simulink model "Resp18e_updatedPulse"  (Simulink 7.3)
settings: Solver=ode23  StartTime=0.0  StopTime=20  FixedStep=0.01  MaxStep=0.05  RelTol=1e-6
values from neighbouring files (symbols this model uses):
  alpha_CO2_brain = 2.9/1e3*760/P_stp/K_stp    (= 0.00097047576489)    [initialize_parameters.m]
  alpha_CO2_fat = 0.9/K_stp/P_stp    (= 0.000396292281489)    [initialize_parameters.m]
  alpha_CO2_heart = 2.4/1e3*760/P_stp/K_stp    (= 0.00080315235715)    [initialize_parameters.m]
  alpha_CO2_lean = 4.2/1e3*760/P_stp/K_stp    (= 0.00140551662501)    [initialize_parameters.m]
  alpha_CO2_lungtiss_fast = alpha_CO2_lungtiss_fast./0.1333    [initialize_parameters.m]
  alpha_CO2_muscle = 4.2/1e3*760/P_stp/K_stp    (= 0.00140551662501)    [initialize_parameters.m]
  alpha_CO2_other = 3.0/1e3*760/P_stp/K_stp    (= 0.00100394044644)    [initialize_parameters.m]
  alpha_O2_fat = 5*0.024/K_stp/P_stp    (= 5.28389708651e-05)    [initialize_parameters.m]
  alpha_O2_tissue = 0.024/K_stp/P_stp    (= 1.0567794173e-05)    [initialize_parameters.m]
  BOHRF0 = O2_SHIFT - T_BLOOD_M_37 * (0.024 + BOHRF * 0.0147) - BOHRF1 * 7.4    (= -3.552)    [initialize_parameters.m]
  BOHRF1 = BOHRF * (1 - T_BLOOD_M_37 * 0.0065)    (= 0.48)    [initialize_parameters.m]
  C_a_CO2_i = 20.8e-3    (= 0.0208)    [initialize_parameters.m]    (also in resp18e_ic_norm.mat = 0.0202734801806)
  C_a_O2_i = 8.95e-3    (= 0.00895)    [initialize_parameters.m]    (also in resp18e_ic_norm.mat = 0.00918087581167)
  CAP_O2 = 0.01 * CAP_O2    (= 0.201)    [initialize_parameters.m]
  Cardiac_duty_cycle = 40    [initialize_parameters.m]
  Co_CO2_brain = 401*K_Co_CO2/1e3/K_stp    (= 0.0107345869894)    [initialize_parameters.m]
  Co_CO2_heart = 487*K_Co_CO2/1e3/K_stp    (= 0.0130367677403)    [initialize_parameters.m]
  Co_CO2_lean = 342*K_Co_CO2/1e3/K_stp    (= 0.00915518391618)    [initialize_parameters.m]
  Co_CO2_muscle = 342*K_Co_CO2/1e3/K_stp    (= 0.00915518391618)    [initialize_parameters.m]
  Co_CO2_other = 355*K_Co_CO2/1e3/K_stp    (= 0.00950318798317)    [initialize_parameters.m]
  DH2ODS = DH2ODS + 0.007 * HB_MEQ * (HB_MEQ - 9) / (13.5 * (13.5 - 9))    (= 0.00498709726946)    [initialize_parameters.m]
  F_insp_alv_alvds = F_v_alv_deadspace / F_insp_hivq    (= 0.00299401197605)    [initialize_parameters.m]
  F_insp_alv_hivq = F_v_alv_hivq      / F_insp_hivq    (= 0.997005988024)    [initialize_parameters.m]
  F_insp_alv_lovq = F_v_alv_lovq      / F_insp_lovq    (= 0.5)    [initialize_parameters.m]
  F_insp_alv_midvq = F_v_alv_midvq     / F_insp_lovq    (= 0.5)    [initialize_parameters.m]
  F_insp_hivq = F_v_alv_deadspace + F_v_alv_hivq    (= 0.334)    [initialize_parameters.m]
  F_insp_lovq = F_v_alv_midvq     + F_v_alv_lovq    (= 0.666)    [initialize_parameters.m]
  Fi_CO2_param_est = 0.01    [initialize_parameters.m]
  Fi_error = 1e-6    (= 1e-06)    [initialize_parameters.m]
  Fi_N2_mean = 1-(Fi_O2_mean + Fi_N2O_mean)    (= 0.65)    [initialize_parameters.m]
  Fi_O2_mean = 0.35    [initialize_parameters.m]
  Fi_O2_param_est = 0.01    [initialize_parameters.m]
  Fq_brain = 0.114    [initialize_parameters.m]
  Fq_error = 1e-8    (= 1e-08)    [initialize_parameters.m]
  Fq_fat = 0.103    [initialize_parameters.m]
  Fq_heart = 0.041    [initialize_parameters.m]
  Fq_hepatic = 0.069    [initialize_parameters.m]
  Fq_kidneys = 0.215    [initialize_parameters.m]
  Fq_lean = 0.090    (= 0.09)    [initialize_parameters.m]
  Fq_lungs_anatomicalshunt = 0.01    [initialize_parameters.m]
  Fq_lungs_hivq = (1-Fq_lungs_pulmshunt-Fq_lungs_anatomicalshunt)    *F_v_alv_hivq/(F_v_alv_hivq+F_v_alv_midvq+F_v_alv_lovq)    (= 0.3)    [initialize_parameters.m]
  Fq_lungs_lovq = (1-Fq_lungs_pulmshunt-Fq_lungs_anatomicalshunt)    *F_v_alv_lovq/(F_v_alv_hivq+F_v_alv_midvq+F_v_alv_lovq)    (= 0.3)    [initialize_parameters.m]
  Fq_lungs_midvq = (1-Fq_lungs_pulmshunt-Fq_lungs_anatomicalshunt)    *F_v_alv_midvq/(F_v_alv_hivq+F_v_alv_midvq+F_v_alv_lovq)    (= 0.3)    [initialize_parameters.m]
  Fq_lungs_pulmshunt = 0.09    [initialize_parameters.m]
  Fq_muscle = 0.096    [initialize_parameters.m]
  Fq_pershunt = 0.101    [initialize_parameters.m]
  Fq_portal = 0.171    [initialize_parameters.m]
  FRC = 2.2    [initialize_parameters.m]
  H2OB = H2OVC + 0.938 * (1 - VC_74)    (= 0.840191964286)    [initialize_parameters.m]
  k_CO2_lungtiss_fast_alvds = k_CO2_lungtiss_fast*F_v_alv_deadspace    (= 3.63090772693e-07)    [initialize_parameters.m]
  k_CO2_lungtiss_fast_hivq = k_CO2_lungtiss_fast*F_v_alv_hivq    (= 0.000120909227307)    [initialize_parameters.m]
  k_CO2_lungtiss_fast_lovq = k_CO2_lungtiss_fast*F_v_alv_lovq    (= 0.000120909227307)    [initialize_parameters.m]
  k_CO2_lungtiss_fast_midvq = k_CO2_lungtiss_fast*F_v_alv_midvq    (= 0.000120909227307)    [initialize_parameters.m]
  k_CO2_lungtiss_slow_alvds = k_CO2_lungtiss_slow*F_v_alv_deadspace    (= 4.95123780945e-09)    [initialize_parameters.m]
  k_CO2_lungtiss_slow_hivq = k_CO2_lungtiss_slow*F_v_alv_hivq    (= 1.64876219055e-06)    [initialize_parameters.m]
  k_CO2_lungtiss_slow_lovq = k_CO2_lungtiss_slow*F_v_alv_lovq    (= 1.64876219055e-06)    [initialize_parameters.m]
  k_CO2_lungtiss_slow_midvq = k_CO2_lungtiss_slow*F_v_alv_midvq    (= 1.64876219055e-06)    [initialize_parameters.m]
  K_diff_CO2_hivq = K_diff_CO2*F_v_alv_hivq    (= 0.0014985)    [initialize_parameters.m]
  K_diff_CO2_lovq = K_diff_CO2*F_v_alv_lovq    (= 0.0014985)    [initialize_parameters.m]
  K_diff_CO2_midvq = K_diff_CO2*F_v_alv_midvq    (= 0.0014985)    [initialize_parameters.m]
  K_diff_O2_hivq = K_diff_O2*F_v_alv_hivq    (= 7.326e-05)    [initialize_parameters.m]
  K_diff_O2_lovq = K_diff_O2*F_v_alv_lovq    (= 7.326e-05)    [initialize_parameters.m]
  K_diff_O2_midvq = K_diff_O2*F_v_alv_midvq    (= 7.326e-05)    [initialize_parameters.m]
  K_exp_alv_alvds = 1/1    (= 1)    [initialize_parameters.m]
  K_exp_alv_hivq = 1/1    (= 1)    [initialize_parameters.m]
  K_press = 760/101.325    (= 7.50061682704)    [initialize_parameters.m]
  K_stp = R*(T_stp+273.15)/(P_stp*1000)    (= 22.4135311621)    [initialize_parameters.m]
  Kg_alv = R*(T_alv+273.15)/(P_baro*1000)    (= 25.3668469802)    [initialize_parameters.m]
  LN10 = 2.30258509299405    (= 2.30258509299)    [initialize_parameters.m]
  m_alv_alvds_i = (FRC-V_deadspace_total)/Kg_alv * F_v_alv_deadspace    [initialize_parameters.m]
  m_alv_hivq_i = (FRC-V_deadspace_total)/Kg_alv * F_v_alv_hivq    [initialize_parameters.m]
  m_alv_lovq_i = (FRC-V_deadspace_total)/Kg_alv * F_v_alv_lovq    [initialize_parameters.m]
  m_alv_midvq_i = (FRC-V_deadspace_total)/Kg_alv * F_v_alv_midvq    [initialize_parameters.m]
  m_CO2_alv_alvds_i = F_CO2_i * m_alv_alvds_i    [initialize_parameters.m]
  m_CO2_alv_hivq_i = F_CO2_i * m_alv_hivq_i    [initialize_parameters.m]
  m_CO2_alv_lovq_i = F_CO2_i * m_alv_lovq_i    [initialize_parameters.m]
  m_CO2_alv_midvq_i = F_CO2_i * m_alv_midvq_i    [initialize_parameters.m]
  m_CO2_brain_b_i = C_a_CO2_i*Vb_brain    (= 0.002184)    [initialize_parameters.m]
  m_CO2_brain_t_i = (Co_CO2_brain  + alpha_CO2_brain *P_v_CO2_i)* Vt_brain    (= 0.0171268217946)    [initialize_parameters.m]
  m_CO2_common_b_i = C_a_CO2_i*Vb_common    (= 0.0170421333333)    [initialize_parameters.m]
  m_CO2_ds0_i = F_CO2_i*m_ds0_i    (= 0.000985538329597)    [initialize_parameters.m]
  m_CO2_ds_large_i = F_CO2_i * m_deadspace_large_1    [initialize_parameters.m]
  m_CO2_ds_med_hivq1_i = F_CO2_i * m_deadspace_med_hivq_1    [initialize_parameters.m]
  m_CO2_ds_med_hivq2_i = F_CO2_i * m_deadspace_med_hivq_2    [initialize_parameters.m]
  m_CO2_ds_med_lovq1_i = F_CO2_i * m_deadspace_med_lovq_1    [initialize_parameters.m]
  m_CO2_ds_med_lovq2_i = F_CO2_i * m_deadspace_med_lovq_2    [initialize_parameters.m]
  m_CO2_ds_small_alvds_i = F_CO2_i * m_deadspace_small_alvdeadspace    [initialize_parameters.m]
  m_CO2_ds_small_hivq_i = F_CO2_i * m_deadspace_small_hivq    [initialize_parameters.m]
  m_CO2_ds_small_lovq_i = F_CO2_i * m_deadspace_small_lovq    [initialize_parameters.m]
  m_CO2_ds_small_midvq_i = F_CO2_i * m_deadspace_small_midvq    [initialize_parameters.m]
  m_CO2_fat_b_i = C_a_CO2_i*Vb_fat    (= 0.0116896)    [initialize_parameters.m]
  m_CO2_fat_t_i = P_a_CO2_i*alpha_CO2_fat*Vt_fat    (= 0.0302752719501)    [initialize_parameters.m]
  m_CO2_heart_b_i = C_a_CO2_i*Vb_heart    (= 0.000832)    [initialize_parameters.m]
  m_CO2_heart_t_i = (Co_CO2_heart  + alpha_CO2_heart *P_v_CO2_i)* Vt_heart    (= 0.00402544335149)    [initialize_parameters.m]
  m_CO2_hepatic_b_i = C_a_CO2_i*Vb_hepatic    (= 0.0019136)    [initialize_parameters.m]
  m_CO2_kidneys_b_i = C_a_CO2_i*Vb_kidneys    (= 0.0012064)    [initialize_parameters.m]
  m_CO2_kidneys_t_i = (Co_CO2_other  + alpha_CO2_other *P_v_CO2_i)* Vt_kidneys    (= 0.0045902552907)    [initialize_parameters.m]
  m_CO2_lean_b_i = C_a_CO2_i*Vb_lean    (= 0.0191984)    [initialize_parameters.m]
  m_CO2_lean_t_i = (Co_CO2_lean   + alpha_CO2_lean  *P_v_CO2_i)* Vt_lean    (= 0.0884995401953)    [initialize_parameters.m]
  m_CO2_liver_t_i = (Co_CO2_other  + alpha_CO2_other *P_v_CO2_i)* Vt_liver    (= 0.0187019339777)    [initialize_parameters.m]
  m_CO2_lungtiss_fast_alvds_i = F_CO2_i*(P_baro-P_A_H2O)*V_lungtiss_alvds *alpha_CO2_lungtiss_fast(2)    [initialize_parameters.m]
  m_CO2_lungtiss_fast_hivq_i = F_CO2_i*(P_baro-P_A_H2O)*V_lungtiss_hivq  *alpha_CO2_lungtiss_fast(2)    [initialize_parameters.m]
  m_CO2_lungtiss_fast_lovq_i = F_CO2_i*(P_baro-P_A_H2O)*V_lungtiss_lovq  *alpha_CO2_lungtiss_fast(2)    [initialize_parameters.m]
  m_CO2_lungtiss_fast_midvq_i = F_CO2_i*(P_baro-P_A_H2O)*V_lungtiss_midvq *alpha_CO2_lungtiss_fast(2)    [initialize_parameters.m]
  m_CO2_lungtiss_slow_alvds_i = F_CO2_i*(P_baro-P_A_H2O)*V_lungtiss_alvds*alpha_CO2_lungtiss_slow    [initialize_parameters.m]
  m_CO2_lungtiss_slow_hivq_i = F_CO2_i*(P_baro-P_A_H2O)*V_lungtiss_hivq *alpha_CO2_lungtiss_slow    [initialize_parameters.m]
  m_CO2_lungtiss_slow_lovq_i = F_CO2_i*(P_baro-P_A_H2O)*V_lungtiss_lovq *alpha_CO2_lungtiss_slow    [initialize_parameters.m]
  m_CO2_lungtiss_slow_midvq_i = F_CO2_i*(P_baro-P_A_H2O)*V_lungtiss_midvq*alpha_CO2_lungtiss_slow    [initialize_parameters.m]
  m_CO2_LV_b_i = C_a_CO2_i*Vb_LV    (= 0.00391733333333)    [initialize_parameters.m]
  m_CO2_muscle_b_i = C_a_CO2_i*Vb_muscle    (= 0.0201344)    [initialize_parameters.m]
  m_CO2_muscle_t_i = (Co_CO2_muscle + alpha_CO2_muscle*P_v_CO2_i)* Vt_muscle    (= 0.363660431061)    [initialize_parameters.m]
  m_CO2_pershunt_b_i = C_a_CO2_i*Vb_pershunt    (= 0.0027248)    [initialize_parameters.m]
  m_CO2_portal_b_i = C_a_CO2_i*Vb_portal    (= 0.0210912)    [initialize_parameters.m]
  m_CO2_portal_t_i = (Co_CO2_other  + alpha_CO2_other *P_v_CO2_i)* Vt_portal    (= 0.0164739329706)    [initialize_parameters.m]
  m_CO2_pulmcap_b_hivq_i = C_a_CO2_i*Vb_pulmcap_hivq    (= 0.000630933333333)    [initialize_parameters.m]
  m_CO2_pulmcap_b_lovq_i = C_a_CO2_i*Vb_pulmcap_lovq    (= 0.000630933333333)    [initialize_parameters.m]
  m_CO2_pulmcap_b_midvq_i = C_a_CO2_i*Vb_pulmcap_midvq    (= 0.000630933333333)    [initialize_parameters.m]
  m_CO2_pulmcap_b_pulmshunt_i = C_a_CO2_i*Vb_pulmcap_pulmshunt    (= 0.0001872)    [initialize_parameters.m]
  m_CO2_RV_b_i = C_v_CO2_i*Vb_RV    (= 0.004181)    [initialize_parameters.m]
  m_N2_alv_alvds_i = Fi_N2_mean * (m_alv_alvds_i - m_CO2_alv_alvds_i)    [initialize_parameters.m]
  ... (+122 more)
undefined symbols (not defined in the file or in its folder): AH2OVC, AHCO3B, DHCO3BDS, litres, mole
libraries: simulink x28
(part 6 of 8)

== system Resp18e_updatedPulse/Patient/Other lean/Lean ==
  note: Note that output vector is C_CO2, C_O2, Fq_heart
  note: NB: Integrators CO2_in and O2_out are purely for mass balance calculations
  note: mole/l
  Ca_gases : Inport  PortDimensions=3  OutDataType=sfix(16)  OutScaling=2^0
  Blood gas curves Olszowka SI Units : Subsystem
  CO2_in : Integrator  InitialConditionSource=external
  CO2_lean : Integrator  InitialCondition=m_CO2_lean_t_i
  C_CO2 body : Gain  Gain=1/Vt_lean  ParameterDataType=sfix(16)  ParameterScaling=2^0  OutDataType=sfix(16)  OutScaling=2^0  SaturateOnIntegerOverflow=on  OutDataTypeStr=Inherit: Same as input  ParamDataTypeStr=Inherit: Same as input
  C_CO2 body1 : Gain  Gain=1/Vt_lean  ParameterDataType=sfix(16)  ParameterScaling=2^0  OutDataType=sfix(16)  OutScaling=2^0  SaturateOnIntegerOverflow=on  OutDataTypeStr=Inherit: Same as input  ParamDataTypeStr=Inherit: Same as input
  C_CO2 body2 : Gain  Gain=-1  ParameterDataType=sfix(16)  ParameterScaling=2^0  OutDataType=sfix(16)  OutScaling=2^0  SaturateOnIntegerOverflow=on  OutDataTypeStr=Inherit: Same as input  ParamDataTypeStr=Inherit: Same as input
  Constant : Constant  Value=0  OutDataType=sfix(16)  OutScaling=2^0
  Constant1 : Constant  Value=0  OutDataType=sfix(16)  OutScaling=2^0
  Demux : Demux  Outputs=3
  InvTissue diss curves : Subsystem
  Mux : Mux  Inputs=3
  O2_lean : Integrator  InitialCondition=m_O2_lean_t_i
  O2_out : Integrator  InitialConditionSource=external
  P4 : Product  Inputs=**  OutDataType=sfix(16)  OutScaling=2^0  SaturateOnIntegerOverflow=on  RndMeth=Zero  InputSameDT=on  OutDataTypeStr=Inherit: Same as first input
  P5 : Product  Inputs=**  OutDataType=sfix(16)  OutScaling=2^0  SaturateOnIntegerOverflow=on  RndMeth=Zero  InputSameDT=on  OutDataTypeStr=Inherit: Same as first input
  P6 : Product  Inputs=**  OutDataType=sfix(16)  OutScaling=2^0  SaturateOnIntegerOverflow=on  RndMeth=Zero  InputSameDT=on  OutDataTypeStr=Inherit: Same as first input
  P_baro1 : Constant  Value=mdot_CO2_lean  OutDataType=sfix(16)  OutScaling=2^0
  P_baro2 : Constant  Value=mdot_O2_lean  OutDataType=sfix(16)  OutScaling=2^0
  Terminator : Terminator
  Terminator1 : Terminator
  Tidal vol2 : Sum  Inputs=-+  OutDataType=sfix(16)  OutScaling=2^0  SaturateOnIntegerOverflow=on  InputSameDT=on  OutDataTypeStr=Inherit: Same as first input
  Tidal vol3 : Sum  Inputs=+-  OutDataType=sfix(16)  OutScaling=2^0  SaturateOnIntegerOverflow=on  InputSameDT=on  OutDataTypeStr=Inherit: Same as first input
  Tidal vol4 : Sum  OutDataType=sfix(16)  OutScaling=2^0  SaturateOnIntegerOverflow=on  InputSameDT=on  OutDataTypeStr=Inherit: Same as first input
  Tidal vol5 : Sum  Inputs=+-  OutDataType=sfix(16)  OutScaling=2^0  SaturateOnIntegerOverflow=on  InputSameDT=on  OutDataTypeStr=Inherit: Same as first input
  To Workspace2 : ToWorkspace  VariableName=C_v_CO2_lean  SampleTime=t_sample  SaveFormat=Array
  To Workspace3 : ToWorkspace  VariableName=C_v_O2_lean  SampleTime=t_sample  SaveFormat=Array
  Cv_gases : Outport  OutDataType=sfix(16)  OutScaling=2^0
  wires:
  Demux/3 -> Mux/3, P6/2
  InvTissue diss curves/2(P_O2) -> Blood gas curves Olszowka SI Units/2(P_O2)
  InvTissue diss curves/1(P_CO2) -> Blood gas curves Olszowka SI Units/1(P_CO2)
  CO2_lean/1 -> C_CO2 body/1
  O2_lean/1 -> C_CO2 body1/1
  [Qpdot] -> P6/1
  P6/1 -> P4/1, P5/1
  Tidal vol5/1 -> O2_lean/1
  P5/1 -> Tidal vol5/1
  P4/1 -> Tidal vol4/2
  Tidal vol4/1 -> CO2_lean/1
  Tidal vol3/1 -> P5/2
  Tidal vol2/1 -> P4/2
  C_CO2 body1/1 -> InvTissue diss curves/2(C_O2)
  C_CO2 body/1 -> InvTissue diss curves/1(C_CO2)
  P_baro1/1 -> Tidal vol4/1, C_CO2 body2/1
  C_CO2 body2/1 -> CO2_in/1
  CO2_in/1 -> Terminator/1
  P_baro2/1 -> Tidal vol5/2, O2_out/1
  O2_out/1 -> Terminator1/1
  Ca_gases/1 -> Demux/1
  Demux/1 -> Tidal vol2/2
  Demux/2 -> Tidal vol3/1
  Mux/1 -> Cv_gases/1
  Blood gas curves Olszowka SI Units/2(C_O2) -> Mux/2, Tidal vol3/2, To Workspace3/1
  Blood gas curves Olszowka SI Units/1(C_CO2) -> Mux/1, Tidal vol2/1, To Workspace2/1
  Constant/1 -> O2_out/2
  Constant1/1 -> CO2_in/2

== system Resp18e_updatedPulse/Patient/Periph Shunt/Delay_pershunt ==
  note: This block performs the following functions:
      | 1. Keeps a record of the quantity of CO2 in aorta
      | 2.  Keeps a record of the quantity of O2 in aorta
      | 3. Delays C_CO2 and C_O2 signals by a time
      | proportional to the aortic volume and inversely
      | proportional to Qpdot.
      | 4. Outputs are delayed C_CO2 and C_O2 signals (moles/l)
      | NB: This subsystem cannot handle varying Qpdot
  note: Constant Qpdot only
  C_gases : Inport  PortDimensions=2  OutDataType=sfix(16)  OutScaling=2^0
  CO2 O2 : Demux  Outputs=2
  CO2 xport delay : VariableTransportDelay  MaximumDelay=20  InitialOutput=C_a_CO2_i  MaximumPoints=n_delay_buffer
  CO2_d : Integrator  InitialCondition=m_CO2_pershunt_b_i
  Fixed delay : Fcn  Expr=Vb_pershunt/u(1)
  Mux : Mux  Inputs=3
  O2 delay : VariableTransportDelay  MaximumDelay=20  InitialOutput=C_a_O2_i  MaximumPoints=n_delay_buffer
  O2_d : Integrator  InitialCondition=m_O2_pershunt_b_i
  Product{1..5} (5 alike) : Product  OutDataType=sfix(16)  OutScaling=2^0  SaturateOnIntegerOverflow=on  RndMeth=Zero  InputSameDT=on  OutDataTypeStr=Inherit: Same as first input
  Terminator : Terminator
  Terminator1 : Terminator
  Tidal vol2 : Sum  Inputs=+-  OutDataType=sfix(16)  OutScaling=2^0  SaturateOnIntegerOverflow=on  InputSameDT=on  OutDataTypeStr=Inherit: Same as first input
  Tidal vol3 : Sum  Inputs=+-  OutDataType=sfix(16)  OutScaling=2^0  SaturateOnIntegerOverflow=on  InputSameDT=on  OutDataTypeStr=Inherit: Same as first input
  Ca_gases_d : Outport  OutDataType=sfix(16)  OutScaling=2^0
  wires:
  [Fq_pershunt] -> Mux/3, Product5/2
  CO2_d/1 -> Terminator1/1
  Fixed delay/1 -> CO2 xport delay/2, O2 delay/2
  Tidal vol2/1 -> CO2_d/1
  Product1/1 -> Tidal vol2/1
  Tidal vol3/1 -> O2_d/1
  Product4/1 -> Tidal vol3/1
  O2_d/1 -> Terminator/1
  CO2 xport delay/1 -> Mux/1, Product2/1
  O2 delay/1 -> Mux/2, Product3/2
  Product3/1 -> Tidal vol3/2
  Product2/1 -> Tidal vol2/2
  CO2 O2/1 -> Product1/1, CO2 xport delay/1
  C_gases/1 -> CO2 O2/1
  CO2 O2/2 -> O2 delay/1, Product4/2
  Mux/1 -> Ca_gases_d/1
  [Qpdot] -> Product5/1
  Product5/1 -> Fixed delay/1, Product1/2, Product3/1, Product4/1, Product2/2

== system Resp18e_updatedPulse/Patient/Pulm cap Hi V/Q/Lung tissue ==
  note: +ve into lung tissue
  note: Lung tissue model after Gronlund (1983) (ref #64)
  PA_CO2 : Inport  OutDataType=sfix(16)  OutScaling=2^0
  CO2_fast : Integrator  Description=Fast tissue compartment  InitialCondition=m_CO2_lungtiss_fast_hivq_i
  CO2_slow : Integrator  InitialCondition=m_CO2_lungtiss_slow_hivq_i
  Gain4 : Gain  Gain=k_CO2_lungtiss_fast_hivq  ParameterDataType=sfix(16)  ParameterScaling=2^0  OutDataType=sfix(16)  OutScaling=2^0  SaturateOnIntegerOverflow=on  OutDataTypeStr=Inherit: Same as input  ParamDataTypeStr=Inherit: Same as input
  Gain5 : Gain  Gain=k_CO2_lungtiss_slow_hivq  ParameterDataType=sfix(16)  ParameterScaling=2^0  OutDataType=sfix(16)  OutScaling=2^0  SaturateOnIntegerOverflow=on  OutDataTypeStr=Inherit: Same as input  ParamDataTypeStr=Inherit: Same as input
  Gain6 : Gain  Gain=1/V_lungtiss_hivq  ParameterDataType=sfix(16)  ParameterScaling=2^0  OutDataType=sfix(16)  OutScaling=2^0  SaturateOnIntegerOverflow=on  OutDataTypeStr=Inherit: Same as input  ParamDataTypeStr=Inherit: Same as input
  Gain7 : Gain  Gain=1/V_lungtiss_hivq/alpha_CO2_lungtiss_slow  ParameterDataType=sfix(16)  ParameterScaling=2^0  OutDataType=sfix(16)  OutScaling=2^0  SaturateOnIntegerOverflow=on  OutDataTypeStr=Inherit: Same as input  ParamDataTypeStr=Inherit: Same as input
  Memory1 : Memory  X0=40*.1333
  P6 : Product  Inputs=*/  OutDataType=sfix(16)  OutScaling=2^0  SaturateOnIntegerOverflow=on  RndMeth=Zero  InputSameDT=on  OutDataTypeStr=Inherit: Same as first input
  alpha_fast1 : Lookup  InputValues=PCO2_alpha  Table=alpha_CO2_lungtiss_fast  OutDataType=sfix(16)  OutScaling=2^0  SaturateOnIntegerOverflow=on
  sum6 : Sum  Inputs=+-  OutDataType=sfix(16)  OutScaling=2^0  SaturateOnIntegerOverflow=on  InputSameDT=on  OutDataTypeStr=Inherit: Same as first input
  sum7 : Sum  Inputs=+-  OutDataType=sfix(16)  OutScaling=2^0  SaturateOnIntegerOverflow=on  InputSameDT=on  OutDataTypeStr=Inherit: Same as first input
  sum8 : Sum  OutDataType=sfix(16)  OutScaling=2^0  SaturateOnIntegerOverflow=on  InputSameDT=on  OutDataTypeStr=Inherit: Same as first input
  mdot_CO2_tissue : Outport  OutDataType=sfix(16)  OutScaling=2^0
  wires:
  sum6/1 -> Gain4/1
  Gain4/1 -> CO2_fast/1, sum8/1
  alpha_fast1/1 -> P6/2
  Memory1/1 -> alpha_fast1/1
  P6/1 -> Memory1/1, sum6/2
  Gain6/1 -> P6/1
  PA_CO2/1 -> sum6/1, sum7/1
  CO2_fast/1 -> Gain6/1
  sum8/1 -> mdot_CO2_tissue/1
  sum7/1 -> Gain5/1
  Gain5/1 -> CO2_slow/1, sum8/2
  CO2_slow/1 -> Gain7/1
  Gain7/1 -> sum7/2

== system Resp18e_updatedPulse/Patient/Pulm cap Hi V/Q/Pulm capillaries ==
  note: This block calculates:
      | 1. The rate of diffusion of CO2 & O2 from the alveolar compartment into the pulmonary capillary blood
      | 2. The resulting CO2 & O2 concentrations in pulmonary capillary blood
      | Note 1: pulm capillary blood becomes arterial blood
      | Note 2: The time constant of this subsystem should remain approx constant as Vb_pulmcap_hivq decreases,
      | becuase Vb_pulmcap_hivq decreases in proportion to Fq_lung_hivq and the loop gain to proportional
      | to Fq_lung_hivq/Vb_pulmcap_hivq.
  note: Pulmonary capillaries
  PA_CO2 : Inport  OutDataType=sfix(16)  OutScaling=2^0
  PA_O2 : Inport  Port=2  OutDataType=sfix(16)  OutScaling=2^0
  C_v_gases : Inport  Port=3  PortDimensions=2  OutDataType=sfix(16)  OutScaling=2^0
  CO2_cap : Integrator  InitialCondition=m_CO2_pulmcap_b_hivq_i
  C_CO2 body : Gain  Gain=1/Vb_pulmcap_hivq  ParameterDataType=sfix(16)  ParameterScaling=2^0  OutDataType=sfix(16)  OutScaling=2^0  SaturateOnIntegerOverflow=on  OutDataTypeStr=Inherit: Same as input  ParamDataTypeStr=Inherit: Same as input
  C_O2 body : Gain  Gain=1/Vb_pulmcap_hivq  ParameterDataType=sfix(16)  ParameterScaling=2^0  OutDataType=sfix(16)  OutScaling=2^0  SaturateOnIntegerOverflow=on  OutDataTypeStr=Inherit: Same as input  ParamDataTypeStr=Inherit: Same as input
  Demux1 : Demux  Outputs=2
  Kdiff_CO2 : Gain  Gain=K_diff_CO2_hivq  ParameterDataType=sfix(16)  ParameterScaling=2^0  OutDataType=sfix(16)  OutScaling=2^0  SaturateOnIntegerOverflow=on  OutDataTypeStr=Inherit: Same as input  ParamDataTypeStr=Inherit: Same as input
  Kdiff_O2 : Gain  Gain=K_diff_O2_hivq  ParameterDataType=sfix(16)  ParameterScaling=2^0  OutDataType=sfix(16)  OutScaling=2^0  SaturateOnIntegerOverflow=on  OutDataTypeStr=Inherit: Same as input  ParamDataTypeStr=Inherit: Same as input
  Mux : Mux  Inputs=2
  Net inflow CO3 : Sum  OutDataType=sfix(16)  OutScaling=2^0  SaturateOnIntegerOverflow=on  InputSameDT=on  OutDataTypeStr=Inherit: Same as first input
  Net inflow CO5 : Sum  Inputs=+-  OutDataType=sfix(16)  OutScaling=2^0  SaturateOnIntegerOverflow=on  InputSameDT=on  OutDataTypeStr=Inherit: Same as first input
  Net inflow CO6 : Sum  Inputs=+-  OutDataType=sfix(16)  OutScaling=2^0  SaturateOnIntegerOverflow=on  InputSameDT=on  OutDataTypeStr=Inherit: Same as first input
  Net inflow CO7 : Sum  OutDataType=sfix(16)  OutScaling=2^0  SaturateOnIntegerOverflow=on  InputSameDT=on  OutDataTypeStr=Inherit: Same as first input
  O2_cap : Integrator  InitialCondition=m_O2_pulmcap_b_hivq_i  AbsoluteTolerance=1e-9
  Olszowka SI units : Subsystem
  P10 : Product  Inputs=**  OutDataType=sfix(16)  OutScaling=2^0  SaturateOnIntegerOverflow=on  RndMeth=Zero  InputSameDT=on  OutDataTypeStr=Inherit: Same as first input
  P8 : Product  Inputs=**  OutDataType=sfix(16)  OutScaling=2^0  SaturateOnIntegerOverflow=on  RndMeth=Zero  InputSameDT=on  OutDataTypeStr=Inherit: Same as first input
  P9 : Product  Inputs=**  OutDataType=sfix(16)  OutScaling=2^0  SaturateOnIntegerOverflow=on  RndMeth=Zero  InputSameDT=on  OutDataTypeStr=Inherit: Same as first input
  Tidal vol4 : Sum  Inputs=-+  OutDataType=sfix(16)  OutScaling=2^0  SaturateOnIntegerOverflow=on  InputSameDT=on  OutDataTypeStr=Inherit: Same as first input
  Tidal vol5 : Sum  Inputs=+-  OutDataType=sfix(16)  OutScaling=2^0  SaturateOnIntegerOverflow=on  InputSameDT=on  OutDataTypeStr=Inherit: Same as first input
  To Workspace3 : ToWorkspace  VariableName=C_ec_hivq_CO2  SampleTime=t_sample  SaveFormat=Array
  To Workspace4 : ToWorkspace  VariableName=C_ec_hivq_O2  SampleTime=t_sample  SaveFormat=Array
  To Workspace6 : ToWorkspace  VariableName=P_ec_hivq_O2  SampleTime=t_sample  SaveFormat=Array
  To Workspace7 : ToWorkspace  VariableName=P_ec_hivq_CO2  SampleTime=t_sample  SaveFormat=Array
  mdot_CO2_A_a : Outport  OutDataType=sfix(16)  OutScaling=2^0
  mdot_O2_A_a : Outport  Port=2  OutDataType=sfix(16)  OutScaling=2^0
  Cec_gases : Outport  Port=3  OutDataType=sfix(16)  OutScaling=2^0
  wires:
  Tidal vol4/1 -> Kdiff_CO2/1
  Olszowka SI units/1(P_CO2) -> Tidal vol4/1, To Workspace7/1
  C_CO2 body/1 -> To Workspace3/1, Olszowka SI units/1(C_CO2), Net inflow CO5/2, Mux/1
  Tidal vol5/1 -> Kdiff_O2/1
  Olszowka SI units/2(P_O2) -> Tidal vol5/2, To Workspace6/1
  Net inflow CO3/1 -> CO2_cap/1
  Kdiff_CO2/1 -> Net inflow CO3/1, mdot_CO2_A_a/1
  P8/1 -> Net inflow CO3/2
  C_O2 body/1 -> To Workspace4/1, Olszowka SI units/2(C_O2), Net inflow CO6/2, Mux/2
  Net inflow CO7/1 -> O2_cap/1
  P9/1 -> Net inflow CO7/2
  CO2_cap/1 -> C_CO2 body/1
  O2_cap/1 -> C_O2 body/1
  Net inflow CO5/1 -> P8/1
  PA_CO2/1 -> Tidal vol4/2  "PA_CO2"
  PA_O2/1 -> Tidal vol5/1  "PAO2"
  Kdiff_O2/1 -> Net inflow CO7/1, mdot_O2_A_a/1
  Demux1/1 -> Net inflow CO5/1
  C_v_gases/1 -> Demux1/1
  Demux1/2 -> Net inflow CO6/1
  Mux/1 -> Cec_gases/1
  Net inflow CO6/1 -> P9/2
  P10/1 -> P8/2, P9/1
  [Qpdot] -> P10/1
  [Fq_lungs_hivq] -> P10/2

== system Resp18e_updatedPulse/Patient/Pulm cap Lo V/Q/Lung tissue ==
  note: +ve into lung tissue
  note: Lung tissue model after Gronlund (1983) (ref #64)
  PA_CO2 : Inport  OutDataType=sfix(16)  OutScaling=2^0
  CO2_fast : Integrator  Description=Fast tissue compartment  InitialCondition=m_CO2_lungtiss_fast_lovq_i
  CO2_slow : Integrator  InitialCondition=m_CO2_lungtiss_slow_lovq_i
  Gain4 : Gain  Gain=k_CO2_lungtiss_fast_lovq  ParameterDataType=sfix(16)  ParameterScaling=2^0  OutDataType=sfix(16)  OutScaling=2^0  SaturateOnIntegerOverflow=on  OutDataTypeStr=Inherit: Same as input  ParamDataTypeStr=Inherit: Same as input
  Gain5 : Gain  Gain=k_CO2_lungtiss_slow_lovq  ParameterDataType=sfix(16)  ParameterScaling=2^0  OutDataType=sfix(16)  OutScaling=2^0  SaturateOnIntegerOverflow=on  OutDataTypeStr=Inherit: Same as input  ParamDataTypeStr=Inherit: Same as input
  Gain6 : Gain  Gain=1/V_lungtiss_lovq  ParameterDataType=sfix(16)  ParameterScaling=2^0  OutDataType=sfix(16)  OutScaling=2^0  SaturateOnIntegerOverflow=on  OutDataTypeStr=Inherit: Same as input  ParamDataTypeStr=Inherit: Same as input
  Gain7 : Gain  Gain=1/V_lungtiss_lovq/alpha_CO2_lungtiss_slow  ParameterDataType=sfix(16)  ParameterScaling=2^0  OutDataType=sfix(16)  OutScaling=2^0  SaturateOnIntegerOverflow=on  OutDataTypeStr=Inherit: Same as input  ParamDataTypeStr=Inherit: Same as input
  Memory1 : Memory  X0=40*.1333
  P6 : Product  Inputs=*/  OutDataType=sfix(16)  OutScaling=2^0  SaturateOnIntegerOverflow=on  RndMeth=Zero  InputSameDT=on  OutDataTypeStr=Inherit: Same as first input
  alpha_fast1 : Lookup  InputValues=PCO2_alpha  Table=alpha_CO2_lungtiss_fast  OutDataType=sfix(16)  OutScaling=2^0  SaturateOnIntegerOverflow=on
  sum6 : Sum  Inputs=+-  OutDataType=sfix(16)  OutScaling=2^0  SaturateOnIntegerOverflow=on  InputSameDT=on  OutDataTypeStr=Inherit: Same as first input
  sum7 : Sum  Inputs=+-  OutDataType=sfix(16)  OutScaling=2^0  SaturateOnIntegerOverflow=on  InputSameDT=on  OutDataTypeStr=Inherit: Same as first input
  sum8 : Sum  OutDataType=sfix(16)  OutScaling=2^0  SaturateOnIntegerOverflow=on  InputSameDT=on  OutDataTypeStr=Inherit: Same as first input
  mdot_CO2_tissue : Outport  OutDataType=sfix(16)  OutScaling=2^0
  wires:
  sum6/1 -> Gain4/1
  Gain4/1 -> CO2_fast/1, sum8/1
  alpha_fast1/1 -> P6/2
  Memory1/1 -> alpha_fast1/1
  P6/1 -> Memory1/1, sum6/2
  Gain6/1 -> P6/1
  PA_CO2/1 -> sum6/1, sum7/1
  CO2_fast/1 -> Gain6/1
  sum8/1 -> mdot_CO2_tissue/1
  sum7/1 -> Gain5/1
  Gain5/1 -> CO2_slow/1, sum8/2
  CO2_slow/1 -> Gain7/1
  Gain7/1 -> sum7/2

== system Resp18e_updatedPulse/Patient/Pulm cap Lo V/Q/Pulm capillaries ==
  note: This block calculates:
      | 1. The rate of diffusion of CO2 & O2 from the alveolar compartment into the pulmonary capillary blood
      | 2. The resulting CO2 & O2 concentrations in pulmonary capillary blood
      | Note: pulm capillary blood becomes arterial blood
  note: Pulmonary capillaries
  PA_CO2 : Inport  OutDataType=sfix(16)  OutScaling=2^0
  PA_O2 : Inport  Port=2  OutDataType=sfix(16)  OutScaling=2^0
  C_v_gases : Inport  Port=3  PortDimensions=2  OutDataType=sfix(16)  OutScaling=2^0
  CO2_cap : Integrator  InitialCondition=m_CO2_pulmcap_b_lovq_i  LimitOutput=on  LowerSaturationLimit=0
  C_CO2 body : Gain  Gain=1/Vb_pulmcap_lovq  ParameterDataType=sfix(16)  ParameterScaling=2^0  OutDataType=sfix(16)  OutScaling=2^0  SaturateOnIntegerOverflow=on  OutDataTypeStr=Inherit: Same as input  ParamDataTypeStr=Inherit: Same as input
  C_O2 body : Gain  Gain=1/Vb_pulmcap_lovq  ParameterDataType=sfix(16)  ParameterScaling=2^0  OutDataType=sfix(16)  OutScaling=2^0  SaturateOnIntegerOverflow=on  OutDataTypeStr=Inherit: Same as input  ParamDataTypeStr=Inherit: Same as input
  Demux1 : Demux  Outputs=2
  Kdiff_CO2 : Gain  Gain=K_diff_CO2_lovq  ParameterDataType=sfix(16)  ParameterScaling=2^0  OutDataType=sfix(16)  OutScaling=2^0  SaturateOnIntegerOverflow=on  OutDataTypeStr=Inherit: Same as input  ParamDataTypeStr=Inherit: Same as input
  Kdiff_O2 : Gain  Gain=K_diff_O2_lovq  ParameterDataType=sfix(16)  ParameterScaling=2^0  OutDataType=sfix(16)  OutScaling=2^0  SaturateOnIntegerOverflow=on  OutDataTypeStr=Inherit: Same as input  ParamDataTypeStr=Inherit: Same as input
  Mux : Mux  Inputs=2
  Net inflow CO3 : Sum  OutDataType=sfix(16)  OutScaling=2^0  SaturateOnIntegerOverflow=on  InputSameDT=on  OutDataTypeStr=Inherit: Same as first input
  Net inflow CO5 : Sum  Inputs=+-  OutDataType=sfix(16)  OutScaling=2^0  SaturateOnIntegerOverflow=on  InputSameDT=on  OutDataTypeStr=Inherit: Same as first input
  Net inflow CO6 : Sum  Inputs=+-  OutDataType=sfix(16)  OutScaling=2^0  SaturateOnIntegerOverflow=on  InputSameDT=on  OutDataTypeStr=Inherit: Same as first input
  Net inflow CO7 : Sum  OutDataType=sfix(16)  OutScaling=2^0  SaturateOnIntegerOverflow=on  InputSameDT=on  OutDataTypeStr=Inherit: Same as first input
  O2_cap : Integrator  InitialCondition=m_O2_pulmcap_b_lovq_i  AbsoluteTolerance=1e-9
  Olszowka SI units : Subsystem
  P10 : Product  Inputs=**  OutDataType=sfix(16)  OutScaling=2^0  SaturateOnIntegerOverflow=on  RndMeth=Zero  InputSameDT=on  OutDataTypeStr=Inherit: Same as first input
  P8 : Product  Inputs=**  OutDataType=sfix(16)  OutScaling=2^0  SaturateOnIntegerOverflow=on  RndMeth=Zero  InputSameDT=on  OutDataTypeStr=Inherit: Same as first input
  P9 : Product  Inputs=**  OutDataType=sfix(16)  OutScaling=2^0  SaturateOnIntegerOverflow=on  RndMeth=Zero  InputSameDT=on  OutDataTypeStr=Inherit: Same as first input
  Tidal vol4 : Sum  Inputs=-+  OutDataType=sfix(16)  OutScaling=2^0  SaturateOnIntegerOverflow=on  InputSameDT=on  OutDataTypeStr=Inherit: Same as first input
  Tidal vol5 : Sum  Inputs=+-  OutDataType=sfix(16)  OutScaling=2^0  SaturateOnIntegerOverflow=on  InputSameDT=on  OutDataTypeStr=Inherit: Same as first input
  To Workspace3 : ToWorkspace  VariableName=C_ec_lovq_CO2  SampleTime=t_sample  SaveFormat=Array
  To Workspace4 : ToWorkspace  VariableName=C_ec_lovq_O2  SampleTime=t_sample  SaveFormat=Array
  To Workspace6 : ToWorkspace  VariableName=P_ec_lovq_O2  SampleTime=t_sample  SaveFormat=Array
  To Workspace7 : ToWorkspace  VariableName=P_ec_lovq_CO2  SampleTime=t_sample  SaveFormat=Array
  mdot_CO2_A_a : Outport  OutDataType=sfix(16)  OutScaling=2^0
  mdot_O2_A_a : Outport  Port=2  OutDataType=sfix(16)  OutScaling=2^0
  Cec_gases : Outport  Port=3  OutDataType=sfix(16)  OutScaling=2^0
  wires:
  Tidal vol4/1 -> Kdiff_CO2/1
  Olszowka SI units/1(P_CO2) -> Tidal vol4/1, To Workspace7/1
  C_CO2 body/1 -> To Workspace3/1, Olszowka SI units/1(C_CO2), Net inflow CO5/2, Mux/1
  Tidal vol5/1 -> Kdiff_O2/1
  Olszowka SI units/2(P_O2) -> Tidal vol5/2, To Workspace6/1
  Net inflow CO3/1 -> CO2_cap/1
  Kdiff_CO2/1 -> Net inflow CO3/1, mdot_CO2_A_a/1
  P8/1 -> Net inflow CO3/2
  C_O2 body/1 -> To Workspace4/1, Olszowka SI units/2(C_O2), Net inflow CO6/2, Mux/2
  Net inflow CO7/1 -> O2_cap/1
  P9/1 -> Net inflow CO7/2
  CO2_cap/1 -> C_CO2 body/1
  O2_cap/1 -> C_O2 body/1
  Net inflow CO5/1 -> P8/1
  PA_CO2/1 -> Tidal vol4/2  "PA_CO2"
  PA_O2/1 -> Tidal vol5/1  "PAO2"
  Kdiff_O2/1 -> Net inflow CO7/1, mdot_O2_A_a/1
  Demux1/1 -> Net inflow CO5/1
  C_v_gases/1 -> Demux1/1
  Demux1/2 -> Net inflow CO6/1
  Mux/1 -> Cec_gases/1
  Net inflow CO6/1 -> P9/2
  P10/1 -> P8/2, P9/1
  [Qpdot] -> P10/1
  [Fq_lungs_lovq] -> P10/2

== system Resp18e_updatedPulse/Patient/Pulm cap Mid V/Q/Lung tissue ==
  note: Lung tissue model after Gronlund (1983) (ref #64)
  note: +ve into lung tissue
  PA_CO2 : Inport  OutDataType=sfix(16)  OutScaling=2^0
  CO2_fast : Integrator  Description=Fast tissue compartment  InitialCondition=m_CO2_lungtiss_fast_midvq_i
  CO2_slow : Integrator  InitialCondition=m_CO2_lungtiss_slow_midvq_i
  Gain4 : Gain  Gain=k_CO2_lungtiss_fast_midvq  ParameterDataType=sfix(16)  ParameterScaling=2^0  OutDataType=sfix(16)  OutScaling=2^0  SaturateOnIntegerOverflow=on  OutDataTypeStr=Inherit: Same as input  ParamDataTypeStr=Inherit: Same as input
  Gain5 : Gain  Gain=k_CO2_lungtiss_slow_midvq  ParameterDataType=sfix(16)  ParameterScaling=2^0  OutDataType=sfix(16)  OutScaling=2^0  SaturateOnIntegerOverflow=on  OutDataTypeStr=Inherit: Same as input  ParamDataTypeStr=Inherit: Same as input
  Gain6 : Gain  Gain=1/V_lungtiss_midvq  ParameterDataType=sfix(16)  ParameterScaling=2^0  OutDataType=sfix(16)  OutScaling=2^0  SaturateOnIntegerOverflow=on  OutDataTypeStr=Inherit: Same as input  ParamDataTypeStr=Inherit: Same as input
  Gain7 : Gain  Gain=1/V_lungtiss_midvq/alpha_CO2_lungtiss_slow  ParameterDataType=sfix(16)  ParameterScaling=2^0  OutDataType=sfix(16)  OutScaling=2^0  SaturateOnIntegerOverflow=on  OutDataTypeStr=Inherit: Same as input  ParamDataTypeStr=Inherit: Same as input
  Memory1 : Memory  X0=40*.1333
  P6 : Product  Inputs=*/  OutDataType=sfix(16)  OutScaling=2^0  SaturateOnIntegerOverflow=on  RndMeth=Zero  InputSameDT=on  OutDataTypeStr=Inherit: Same as first input
  To Workspace18 : ToWorkspace  VariableName=mdot_CO2_tissue_fast_midvq  SampleTime=t_sample  SaveFormat=Array
  To Workspace19 : ToWorkspace  VariableName=mdot_CO2_tissue_slow_midvq  SampleTime=t_sample  SaveFormat=Array
  To Workspace20 : ToWorkspace  VariableName=m_CO2_tissue_fast_midvq  SampleTime=t_sample  SaveFormat=Array
  To Workspace21 : ToWorkspace  VariableName=m_CO2_tissue_slow_midvq  SampleTime=t_sample  SaveFormat=Array
  alpha_fast1 : Lookup  InputValues=PCO2_alpha  Table=alpha_CO2_lungtiss_fast  OutDataType=sfix(16)  OutScaling=2^0  SaturateOnIntegerOverflow=on
  sum6 : Sum  Inputs=+-  OutDataType=sfix(16)  OutScaling=2^0  SaturateOnIntegerOverflow=on  InputSameDT=on  OutDataTypeStr=Inherit: Same as first input
  sum7 : Sum  Inputs=+-  OutDataType=sfix(16)  OutScaling=2^0  SaturateOnIntegerOverflow=on  InputSameDT=on  OutDataTypeStr=Inherit: Same as first input
  sum8 : Sum  OutDataType=sfix(16)  OutScaling=2^0  SaturateOnIntegerOverflow=on  InputSameDT=on  OutDataTypeStr=Inherit: Same as first input
  mdot_CO2_tissue : Outport  OutDataType=sfix(16)  OutScaling=2^0
  wires:
  Gain7/1 -> sum7/2
  Gain5/1 -> CO2_slow/1, sum8/2, To Workspace19/1
  sum7/1 -> Gain5/1
  sum8/1 -> mdot_CO2_tissue/1
  PA_CO2/1 -> sum7/1, sum6/1
  Gain6/1 -> P6/1
  P6/1 -> sum6/2, Memory1/1
  Memory1/1 -> alpha_fast1/1
  alpha_fast1/1 -> P6/2
  Gain4/1 -> CO2_fast/1, sum8/1, To Workspace18/1
  sum6/1 -> Gain4/1
  CO2_fast/1 -> Gain6/1, To Workspace20/1
  CO2_slow/1 -> Gain7/1, To Workspace21/1

== system Resp18e_updatedPulse/Patient/Pulm cap Mid V/Q/Pulm capillaries ==
  note: Pulmonary capillaries
  note: This block calculates:
      | 1. The rate of diffusion of CO2 & O2 from the alveolar compartment into the pulmonary capillary blood
      | 2. The resulting CO2 & O2 concentrations in pulmonary capillary blood
      | Note: pulm capillary blood becomes arterial blood
  PA_CO2 : Inport  OutDataType=sfix(16)  OutScaling=2^0
  PA_O2 : Inport  Port=2  OutDataType=sfix(16)  OutScaling=2^0
  C_v_gases : Inport  Port=3  PortDimensions=2  OutDataType=sfix(16)  OutScaling=2^0
  CO2_cap : Integrator  InitialCondition=m_CO2_pulmcap_b_midvq_i
  C_CO2 body : Gain  Gain=1/Vb_pulmcap_midvq  ParameterDataType=sfix(16)  ParameterScaling=2^0  OutDataType=sfix(16)  OutScaling=2^0  SaturateOnIntegerOverflow=on  OutDataTypeStr=Inherit: Same as input  ParamDataTypeStr=Inherit: Same as input
  C_O2 body : Gain  Gain=1/Vb_pulmcap_midvq  ParameterDataType=sfix(16)  ParameterScaling=2^0  OutDataType=sfix(16)  OutScaling=2^0  SaturateOnIntegerOverflow=on  OutDataTypeStr=Inherit: Same as input  ParamDataTypeStr=Inherit: Same as input
  Demux1 : Demux  Outputs=2
  Kdiff_CO2 : Gain  Gain=K_diff_CO2_midvq  ParameterDataType=sfix(16)  ParameterScaling=2^0  OutDataType=sfix(16)  OutScaling=2^0  SaturateOnIntegerOverflow=on  OutDataTypeStr=Inherit: Same as input  ParamDataTypeStr=Inherit: Same as input
  Kdiff_O2 : Gain  Gain=K_diff_O2_midvq  ParameterDataType=sfix(16)  ParameterScaling=2^0  OutDataType=sfix(16)  OutScaling=2^0  SaturateOnIntegerOverflow=on  OutDataTypeStr=Inherit: Same as input  ParamDataTypeStr=Inherit: Same as input
  Mux : Mux  Inputs=2
  Net inflow CO3 : Sum  OutDataType=sfix(16)  OutScaling=2^0  SaturateOnIntegerOverflow=on  InputSameDT=on  OutDataTypeStr=Inherit: Same as first input
  Net inflow CO5 : Sum  Inputs=+-  OutDataType=sfix(16)  OutScaling=2^0  SaturateOnIntegerOverflow=on  InputSameDT=on  OutDataTypeStr=Inherit: Same as first input
  Net inflow CO6 : Sum  Inputs=+-  OutDataType=sfix(16)  OutScaling=2^0  SaturateOnIntegerOverflow=on  InputSameDT=on  OutDataTypeStr=Inherit: Same as first input
  Net inflow CO7 : Sum  OutDataType=sfix(16)  OutScaling=2^0  SaturateOnIntegerOverflow=on  InputSameDT=on  OutDataTypeStr=Inherit: Same as first input
  O2_cap : Integrator  InitialCondition=m_O2_pulmcap_b_midvq_i  AbsoluteTolerance=1e-9
  Olszowka SI units : Subsystem
  P10 : Product  Inputs=**  OutDataType=sfix(16)  OutScaling=2^0  SaturateOnIntegerOverflow=on  RndMeth=Zero  InputSameDT=on  OutDataTypeStr=Inherit: Same as first input
  P8 : Product  Inputs=**  OutDataType=sfix(16)  OutScaling=2^0  SaturateOnIntegerOverflow=on  RndMeth=Zero  InputSameDT=on  OutDataTypeStr=Inherit: Same as first input
  P9 : Product  Inputs=**  OutDataType=sfix(16)  OutScaling=2^0  SaturateOnIntegerOverflow=on  RndMeth=Zero  InputSameDT=on  OutDataTypeStr=Inherit: Same as first input
  Tidal vol4 : Sum  Inputs=-+  OutDataType=sfix(16)  OutScaling=2^0  SaturateOnIntegerOverflow=on  InputSameDT=on  OutDataTypeStr=Inherit: Same as first input
  Tidal vol5 : Sum  Inputs=+-  OutDataType=sfix(16)  OutScaling=2^0  SaturateOnIntegerOverflow=on  InputSameDT=on  OutDataTypeStr=Inherit: Same as first input
  To Workspace3 : ToWorkspace  VariableName=C_ec_midvq_CO2  SampleTime=t_sample  SaveFormat=Array
  To Workspace4 : ToWorkspace  VariableName=C_ec_midvq_O2  SampleTime=t_sample  SaveFormat=Array
  To Workspace6 : ToWorkspace  VariableName=P_ec_midvq_O2  SampleTime=t_sample  SaveFormat=Array
  To Workspace7 : ToWorkspace  VariableName=P_ec_midvq_CO2  SampleTime=t_sample  SaveFormat=Array
  mdot_CO2_A_a : Outport  OutDataType=sfix(16)  OutScaling=2^0
  mdot_O2_A_a : Outport  Port=2  OutDataType=sfix(16)  OutScaling=2^0
  Cec_gases : Outport  Port=3  OutDataType=sfix(16)  OutScaling=2^0
  wires:
  [Qpdot] -> P10/1
  P10/1 -> P9/1, P8/2
  Net inflow CO6/1 -> P9/2
  Mux/1 -> Cec_gases/1
  Demux1/2 -> Net inflow CO6/1
  C_v_gases/1 -> Demux1/1
  Demux1/1 -> Net inflow CO5/1
  Kdiff_O2/1 -> mdot_O2_A_a/1, Net inflow CO7/1
  PA_O2/1 -> Tidal vol5/1  "PAO2"
  PA_CO2/1 -> Tidal vol4/2  "PA_CO2"
  Net inflow CO5/1 -> P8/1
  O2_cap/1 -> C_O2 body/1
  CO2_cap/1 -> C_CO2 body/1
  P9/1 -> Net inflow CO7/2
  Net inflow CO7/1 -> O2_cap/1
  C_O2 body/1 -> Mux/2, Net inflow CO6/2, Olszowka SI units/2(C_O2), To Workspace4/1
  P8/1 -> Net inflow CO3/2
  Kdiff_CO2/1 -> mdot_CO2_A_a/1, Net inflow CO3/1
  Net inflow CO3/1 -> CO2_cap/1
  Olszowka SI units/2(P_O2) -> To Workspace6/1, Tidal vol5/2
  Tidal vol5/1 -> Kdiff_O2/1
  C_CO2 body/1 -> Mux/1, Net inflow CO5/2, Olszowka SI units/1(C_CO2), To Workspace3/1
  Olszowka SI units/1(P_CO2) -> To Workspace7/1, Tidal vol4/1
  Tidal vol4/1 -> Kdiff_CO2/1
  [Fq_lungs_midvq] -> P10/2

== system Resp18e_updatedPulse/Patient/Anaesthetic Machine & resp mechanics/Insp gas mixing/Insp gas calcs ==
  note: WK: removed pole cancel blocks
  CO2 Resp PWM : Subsystem
  FiN2O+FiN2O : Constant  Value=Fi_O2_mean  OutDataType=sfix(16)  OutScaling=2^0
  Gain1 : Gain  Gain=Fi_CO2_param_est  ParameterDataType=sfix(16)  ParameterScaling=2^0  OutDataType=sfix(16)  OutScaling=2^0  SaturateOnIntegerOverflow=on  OutDataTypeStr=Inherit: Same as input  ParamDataTypeStr=Inherit: Same as input
  Gain2 : Gain  Gain=Fi_O2_param_est  ParameterDataType=sfix(16)  ParameterScaling=2^0  OutDataType=sfix(16)  OutScaling=2^0  SaturateOnIntegerOverflow=on  OutDataTypeStr=Inherit: Same as input  ParamDataTypeStr=Inherit: Same as input
  Limits : Saturate  UpperLimit=1  LowerLimit=0
  Limits1 : Saturate  UpperLimit=1  LowerLimit=0
  Mean FiN2 : Constant  Value=Fi_N2_mean  OutDataType=sfix(16)  OutScaling=2^0
  Mean FiN3 : Constant  Value=0  OutDataType=sfix(16)  OutScaling=2^0
  Mean FiN4 : Constant  Value=0  OutDataType=sfix(16)  OutScaling=2^0
  Pulse Generator : DiscretePulseGenerator  PulseType=Time based  Amplitude=1  Period=T_pulse_repeat  PulseWidth=pulse_duty_cycle  PhaseDelay=T_pulse_start  SampleTime=1
  Switch2 : Switch  Threshold=.5  SaturateOnIntegerOverflow=on  InputSameDT=on
  Switch3 : Switch  Threshold=.5  SaturateOnIntegerOverflow=on  InputSameDT=on
  a : Sum  OutDataType=sfix(16)  OutScaling=2^0  SaturateOnIntegerOverflow=on  InputSameDT=on  OutDataTypeStr=Inherit: Same as first input
  a1 : Sum  OutDataType=sfix(16)  OutScaling=2^0  SaturateOnIntegerOverflow=on  InputSameDT=on  OutDataTypeStr=Inherit: Same as first input
  b : Sum  Inputs=-+  OutDataType=sfix(16)  OutScaling=2^0  SaturateOnIntegerOverflow=on  InputSameDT=on  OutDataTypeStr=Inherit: Same as first input
  Fi_O2 : Outport  OutDataType=sfix(16)  OutScaling=2^0
  Fi_CO2 : Outport  Port=2  OutDataType=sfix(16)  OutScaling=2^0
  Fi_N2 : Outport  Port=3  OutDataType=sfix(16)  OutScaling=2^0
  wires:
  CO2 Resp PWM/1(Out1) -> Switch2/2, Switch3/2
  FiN2O+FiN2O/1 -> a/1
  Mean FiN2/1 -> b/2
  b/1 -> Fi_N2/1
  Mean FiN3/1 -> Switch2/3
  a/1 -> Fi_O2/1
  Mean FiN4/1 -> Switch3/3
  Switch2/1 -> a1/1, Fi_CO2/1
  Switch3/1 -> a/2, a1/2
  a1/1 -> b/1
  Pulse Generator/1 -> Gain2/1, Gain1/1
  Limits1/1 -> Switch3/1
  Limits/1 -> Switch2/1
  Gain1/1 -> Limits/1
  Gain2/1 -> Limits1/1

== system Resp18e_updatedPulse/Patient/Brain/Brain/Blood gas curves Olszowka SI Units ==
  P_CO2 : Inport  OutDataType=sfix(16)  OutScaling=2^0
  P_O2 : Inport  Port=2  OutDataType=sfix(16)  OutScaling=2^0
  Olszowka's diss curves : Subsystem
  kPa > mm Hg : Gain  Gain=K_press  ParameterDataType=sfix(16)  ParameterScaling=2^0  OutDataType=sfix(16)  OutScaling=2^0  SaturateOnIntegerOverflow=on  OutDataTypeStr=Inherit: Same as input  ParamDataTypeStr=Inherit: Same as input
  kPa > mm Hg1 : Gain  Gain=K_press  ParameterDataType=sfix(16)  ParameterScaling=2^0  OutDataType=sfix(16)  OutScaling=2^0  SaturateOnIntegerOverflow=on  OutDataTypeStr=Inherit: Same as input  ParamDataTypeStr=Inherit: Same as input
  l > mole : Gain  Gain=1/K_stp  ParameterDataType=sfix(16)  ParameterScaling=2^0  OutDataType=sfix(16)  OutScaling=2^0  SaturateOnIntegerOverflow=on  OutDataTypeStr=Inherit: Same as input  ParamDataTypeStr=Inherit: Same as input
  l> mole : Gain  Gain=1/K_stp  ParameterDataType=sfix(16)  ParameterScaling=2^0  OutDataType=sfix(16)  OutScaling=2^0  SaturateOnIntegerOverflow=on  OutDataTypeStr=Inherit: Same as input  ParamDataTypeStr=Inherit: Same as input
  C_CO2 : Outport  OutDataType=sfix(16)  OutScaling=2^0
  C_O2 : Outport  Port=2  OutDataType=sfix(16)  OutScaling=2^0
  wires:
  kPa > mm Hg/1 -> Olszowka's diss curves/1(P_CO2)
  kPa > mm Hg1/1 -> Olszowka's diss curves/2(PO2)
  Olszowka's diss curves/1(C_CO2) -> l > mole/1
  Olszowka's diss curves/2(C_O2) -> l> mole/1
  l > mole/1 -> C_CO2/1
  P_CO2/1 -> kPa > mm Hg/1
  l> mole/1 -> C_O2/1
  P_O2/1 -> kPa > mm Hg1/1

== system Resp18e_updatedPulse/Patient/Brain/Brain/InvTissue diss curves ==
  note: mole/l
  note: kPa
  C_CO2 : Inport  OutDataType=sfix(16)  OutScaling=2^0
  C_O2 : Inport  Port=2  OutDataType=sfix(16)  OutScaling=2^0
  q : Fcn  Expr=u(1)/alpha_O2_tissue
  q1 : Fcn  Expr=(u(1)-Co_CO2_brain)/alpha_CO2_brain
  PT_CO2 : Outport  OutDataType=sfix(16)  OutScaling=2^0
  PT_O2 : Outport  Port=2  OutDataType=sfix(16)  OutScaling=2^0
  wires:
  C_O2/1 -> q/1
  q/1 -> PT_O2/1  "PO2"
  C_CO2/1 -> q1/1
  q1/1 -> PT_CO2/1  "PCO2"

== system Resp18e_updatedPulse/Patient/Fat/fat/Blood gas curves Olszowka SI Units ==
  P_CO2 : Inport  OutDataType=sfix(16)  OutScaling=2^0
  P_O2 : Inport  Port=2  OutDataType=sfix(16)  OutScaling=2^0
  Olszowka's diss curves : Subsystem
  kPa > mm Hg : Gain  Gain=K_press  ParameterDataType=sfix(16)  ParameterScaling=2^0  OutDataType=sfix(16)  OutScaling=2^0  SaturateOnIntegerOverflow=on  OutDataTypeStr=Inherit: Same as input  ParamDataTypeStr=Inherit: Same as input
  kPa > mm Hg1 : Gain  Gain=K_press  ParameterDataType=sfix(16)  ParameterScaling=2^0  OutDataType=sfix(16)  OutScaling=2^0  SaturateOnIntegerOverflow=on  OutDataTypeStr=Inherit: Same as input  ParamDataTypeStr=Inherit: Same as input
  l > mole : Gain  Gain=1/K_stp  ParameterDataType=sfix(16)  ParameterScaling=2^0  OutDataType=sfix(16)  OutScaling=2^0  SaturateOnIntegerOverflow=on  OutDataTypeStr=Inherit: Same as input  ParamDataTypeStr=Inherit: Same as input
  l> mole : Gain  Gain=1/K_stp  ParameterDataType=sfix(16)  ParameterScaling=2^0  OutDataType=sfix(16)  OutScaling=2^0  SaturateOnIntegerOverflow=on  OutDataTypeStr=Inherit: Same as input  ParamDataTypeStr=Inherit: Same as input
  C_CO2 : Outport  OutDataType=sfix(16)  OutScaling=2^0
  C_O2 : Outport  Port=2  OutDataType=sfix(16)  OutScaling=2^0
  wires:
  kPa > mm Hg/1 -> Olszowka's diss curves/1(P_CO2)
  kPa > mm Hg1/1 -> Olszowka's diss curves/2(PO2)
  Olszowka's diss curves/1(C_CO2) -> l > mole/1
  Olszowka's diss curves/2(C_O2) -> l> mole/1
  l > mole/1 -> C_CO2/1
  P_CO2/1 -> kPa > mm Hg/1
  l> mole/1 -> C_O2/1
  P_O2/1 -> kPa > mm Hg1/1

== system Resp18e_updatedPulse/Patient/Fat/fat/Inv fat diss curves ==
  note: mole/l
  note: mole/l
  note: kPa
  note: kPa
  C_CO2 : Inport  OutDataType=sfix(16)  OutScaling=2^0
  C_O2 : Inport  Port=2  OutDataType=sfix(16)  OutScaling=2^0
  fat : Fcn  Expr=u(1)/alpha_CO2_fat
  fat1 : Fcn  Expr=u(1)/alpha_O2_fat
  P_CO2 : Outport  OutDataType=sfix(16)  OutScaling=2^0
  P_O2 : Outport  Port=2  OutDataType=sfix(16)  OutScaling=2^0
  wires:
  C_O2/1 -> fat1/1
  fat1/1 -> P_O2/1  "PTO2"
  C_CO2/1 -> fat/1
  fat/1 -> P_CO2/1  "PTCO2"

== system Resp18e_updatedPulse/Patient/Heart/Heart/Blood gas curves Olszowka SI Units ==
  P_CO2 : Inport  OutDataType=sfix(16)  OutScaling=2^0
  P_O2 : Inport  Port=2  OutDataType=sfix(16)  OutScaling=2^0
  Olszowka's diss curves : Subsystem
  kPa > mm Hg : Gain  Gain=K_press  ParameterDataType=sfix(16)  ParameterScaling=2^0  OutDataType=sfix(16)  OutScaling=2^0  SaturateOnIntegerOverflow=on  OutDataTypeStr=Inherit: Same as input  ParamDataTypeStr=Inherit: Same as input
  kPa > mm Hg1 : Gain  Gain=K_press  ParameterDataType=sfix(16)  ParameterScaling=2^0  OutDataType=sfix(16)  OutScaling=2^0  SaturateOnIntegerOverflow=on  OutDataTypeStr=Inherit: Same as input  ParamDataTypeStr=Inherit: Same as input
  l > mole : Gain  Gain=1/K_stp  ParameterDataType=sfix(16)  ParameterScaling=2^0  OutDataType=sfix(16)  OutScaling=2^0  SaturateOnIntegerOverflow=on  OutDataTypeStr=Inherit: Same as input  ParamDataTypeStr=Inherit: Same as input
  l> mole : Gain  Gain=1/K_stp  ParameterDataType=sfix(16)  ParameterScaling=2^0  OutDataType=sfix(16)  OutScaling=2^0  SaturateOnIntegerOverflow=on  OutDataTypeStr=Inherit: Same as input  ParamDataTypeStr=Inherit: Same as input
  C_CO2 : Outport  OutDataType=sfix(16)  OutScaling=2^0
  C_O2 : Outport  Port=2  OutDataType=sfix(16)  OutScaling=2^0
  wires:
  kPa > mm Hg/1 -> Olszowka's diss curves/1(P_CO2)
  kPa > mm Hg1/1 -> Olszowka's diss curves/2(PO2)
  Olszowka's diss curves/1(C_CO2) -> l > mole/1
  Olszowka's diss curves/2(C_O2) -> l> mole/1
  l > mole/1 -> C_CO2/1
  P_CO2/1 -> kPa > mm Hg/1
  l> mole/1 -> C_O2/1
  P_O2/1 -> kPa > mm Hg1/1

== system Resp18e_updatedPulse/Patient/Heart/Heart/InvTissue diss curves ==
  note: mole/l
  note: kPa
  C_CO2 : Inport  OutDataType=sfix(16)  OutScaling=2^0
  C_O2 : Inport  Port=2  OutDataType=sfix(16)  OutScaling=2^0
  q : Fcn  Expr=u(1)/alpha_O2_tissue
  q1 : Fcn  Expr=(u(1)-Co_CO2_heart)/alpha_CO2_heart
  PT_CO2 : Outport  OutDataType=sfix(16)  OutScaling=2^0
  PT_O2 : Outport  Port=2  OutDataType=sfix(16)  OutScaling=2^0
  wires:
  C_O2/1 -> q/1
  q/1 -> PT_O2/1  "PO2"
  C_CO2/1 -> q1/1
  q1/1 -> PT_CO2/1  "PCO2"
